simulink model "Braccio_trajectory_tracking_signal_based"  (R2021a)
settings: Solver=FixedStepAuto  StartTime=0.0  StopTime=inf  RelTol=1e-3  EnableMultiTasking=on
InitFcn:
  | cBase=90;
  | cShoulder=90;
  | cElbow=90;
  | cWristVer=90;
  | cWristRot=90;
  | cGripper=73;
undefined symbols (not defined in the file or in its folder): sigbuilder_block
libraries: arduinolib x7, simulink x1, sldrtlib x1
settings Model: SILPILModeSetting=veronly  ExtModeTrigDuration=2  Creator=loris  LastModifiedBy=loris
settings OptimizationCC: EnhancedBackFolding=on  PassReuseOutputArgsAs=Individual arguments  ZeroExternalMemoryAtStartup=off  ZeroInternalMemoryAtStartup=off  MaxStackSize=64  OptimizeBlockOrder=speed  DifferentSizesBufferReuse=on  OptimizationCustomize=off  EfficientTunableParamExpr=on
settings DebuggingCC: ParameterTunabilityLossMsg=error
settings HardwareCC: ProdBitPerInt=16  ProdBitPerPointer=16  ProdBitPerSizeT=16  ProdBitPerPtrDiffT=16  ProdLargestAtomicFloat=None  ProdWordSize=8  ProdHWDeviceType=Atmel->AVR
settings SFSimCC: MATLABDynamicMemAlloc=off
settings RTWCC: SystemTargetFile=ert.tlc  HardwareBoard=Arduino Mega 2560  TemplateMakefile=ert_default_tmf  Toolchain=Arduino AVR  BuildConfiguration=Faster Runs
settings CodeAppCC: ForceParamTrailComments=on  IgnoreCustomStorageClasses=off  OperatorAnnotations=on  SimulinkDataObjDesc=on  SFDataObjDesc=on  InsertBlockDesc=on
settings ERTTargetCC: SupportContinuousTime=on  SupportVariableSizeSignals=on  ExtModeStaticAllocSize=2048

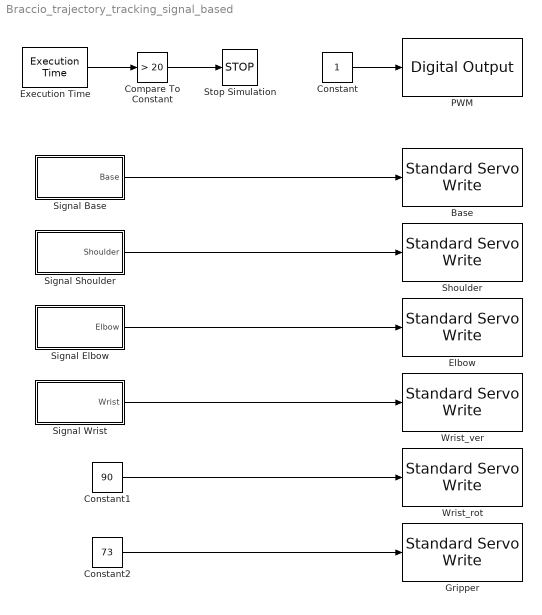
== system Braccio_trajectory_tracking_signal_based ==
  Base : arduinolib/Standard Servo Write  pinNumber=11  ServoIndex=0  blockPlatform=ARDUINO
  Compare To Constant : simulink/Logic and Bit Operations/Compare To Constant  relop=>  const=20  OutDataTypeStr=boolean
  Constant : Constant
  Constant1 : Constant  Value=90
  Constant2 : Constant  Value=73
  Elbow : arduinolib/Standard Servo Write  pinNumber=9  ServoIndex=1  blockPlatform=ARDUINO
  Execution Time : sldrtlib/Target Profiling/Execution Time  ShowTaskTimes=off
      settings: SourceProductBaseCode=WT
  Gripper : arduinolib/Standard Servo Write  pinNumber=3  ServoIndex=2  blockPlatform=ARDUINO
  PWM : arduinolib/Digital Output  pinNumber=12  Direction=output  blockPlatform=arduino
  Shoulder : arduinolib/Standard Servo Write  pinNumber=10  ServoIndex=3  blockPlatform=ARDUINO
  Signal Base : Subsystem  Tag=STV Subsys  LoadFcn=sigbuilder_block('load');  StartFcn=sigbuilder_block('start');  StopFcn=sigbuilder_block('stop');  ClipboardFcn=sigbuilder_block('clipboard');  mask(Sigbuilder block){tuvar=[0:10]}
      mask help: Simulink:masks:SigbuilderBlock_MD
      mask init:
      | if ~strcmp(get_param(bdroot(gcbh),'SimulationStatus'),'stopped') tuvar = sigbuilder_block('maskInit'); end
      settings: CopyFcn=sigbuilder_block('copy');  DeleteFcn=sigbuilder_block('delete');  ModelCloseFcn=sigbuilder_block('modelClose');  PreSaveFcn=sigbuilder_block('preSave');  PauseFcn=sigbuilder_block('pause');  ContinueFcn=sigbuilder_block('continue');  NameChangeFcn=sigbuilder_block('namechange');  OpenFcn=sigbuilder_block('open',[594 1310 550 349 ]);  CloseFcn=sigbuilder_block('close');
      mask Display: plot(0, 0, 100, 100,[2, 2, 32, 32, 2], [68, 8, 8, 68, 68],[32, 2], [38, 38], [32, 19, 2],[53, 60, 44], [32, 17, 17, 2],[16, 16, 31, 31]);txt = getActiveGroup(gcbh);text(2, 100, txt,'verticalAlignment', 'top');
  Signal Elbow : Subsystem  Tag=STV Subsys  LoadFcn=sigbuilder_block('load');  StartFcn=sigbuilder_block('start');  StopFcn=sigbuilder_block('stop');  ClipboardFcn=sigbuilder_block('clipboard');  mask(Sigbuilder block){tuvar=[0:10]}
      mask help: Simulink:masks:SigbuilderBlock_MD
      mask init:
      | if ~strcmp(get_param(bdroot(gcbh),'SimulationStatus'),'stopped') tuvar = sigbuilder_block('maskInit'); end
      settings: CopyFcn=sigbuilder_block('copy');  DeleteFcn=sigbuilder_block('delete');  ModelCloseFcn=sigbuilder_block('modelClose');  PreSaveFcn=sigbuilder_block('preSave');  PauseFcn=sigbuilder_block('pause');  ContinueFcn=sigbuilder_block('continue');  NameChangeFcn=sigbuilder_block('namechange');  OpenFcn=sigbuilder_block('open',[437.6 199.2 550.4 400 ]);  CloseFcn=sigbuilder_block('close');
      mask Display: plot(0, 0, 100, 100,[2, 2, 32, 32, 2], [68, 8, 8, 68, 68],[32, 2], [38, 38], [32, 19, 2],[53, 60, 44], [32, 17, 17, 2],[16, 16, 31, 31]);txt = getActiveGroup(gcbh);text(2, 100, txt,'verticalAlignment', 'top');
  Signal Shoulder : Subsystem  Tag=STV Subsys  LoadFcn=sigbuilder_block('load');  StartFcn=sigbuilder_block('start');  StopFcn=sigbuilder_block('stop');  ClipboardFcn=sigbuilder_block('clipboard');  mask(Sigbuilder block){tuvar=[0:10]}
      mask help: Simulink:masks:SigbuilderBlock_MD
      mask init:
      | if ~strcmp(get_param(bdroot(gcbh),'SimulationStatus'),'stopped') tuvar = sigbuilder_block('maskInit'); end
      settings: CopyFcn=sigbuilder_block('copy');  DeleteFcn=sigbuilder_block('delete');  ModelCloseFcn=sigbuilder_block('modelClose');  PreSaveFcn=sigbuilder_block('preSave');  PauseFcn=sigbuilder_block('pause');  ContinueFcn=sigbuilder_block('continue');  NameChangeFcn=sigbuilder_block('namechange');  OpenFcn=sigbuilder_block('open',[585 316 550 400 ]);  CloseFcn=sigbuilder_block('close');
      mask Display: plot(0, 0, 100, 100,[2, 2, 32, 32, 2], [68, 8, 8, 68, 68],[32, 2], [38, 38], [32, 19, 2],[53, 60, 44], [32, 17, 17, 2],[16, 16, 31, 31]);txt = getActiveGroup(gcbh);text(2, 100, txt,'verticalAlignment', 'top');
  Signal Wrist : Subsystem  Tag=STV Subsys  LoadFcn=sigbuilder_block('load');  StartFcn=sigbuilder_block('start');  StopFcn=sigbuilder_block('stop');  ClipboardFcn=sigbuilder_block('clipboard');  mask(Sigbuilder block){tuvar=[0:10]}
      mask help: Simulink:masks:SigbuilderBlock_MD
      mask init:
      | if ~strcmp(get_param(bdroot(gcbh),'SimulationStatus'),'stopped') tuvar = sigbuilder_block('maskInit'); end
      settings: CopyFcn=sigbuilder_block('copy');  DeleteFcn=sigbuilder_block('delete');  ModelCloseFcn=sigbuilder_block('modelClose');  PreSaveFcn=sigbuilder_block('preSave');  PauseFcn=sigbuilder_block('pause');  ContinueFcn=sigbuilder_block('continue');  NameChangeFcn=sigbuilder_block('namechange');  OpenFcn=sigbuilder_block('open',[437.6 199.2 550.4 400 ]);  CloseFcn=sigbuilder_block('close');
      mask Display: plot(0, 0, 100, 100,[2, 2, 32, 32, 2], [68, 8, 8, 68, 68],[32, 2], [38, 38], [32, 19, 2],[53, 60, 44], [32, 17, 17, 2],[16, 16, 31, 31]);txt = getActiveGroup(gcbh);text(2, 100, txt,'verticalAlignment', 'top');
  Stop Simulation : Stop
  Wrist_rot : arduinolib/Standard Servo Write  pinNumber=5  ServoIndex=4  blockPlatform=ARDUINO
  Wrist_ver : arduinolib/Standard Servo Write  pinNumber=6  ServoIndex=5  blockPlatform=ARDUINO
  wires:
  Constant/1 -> PWM/1
  Signal Base/1(Base) -> Base/1
  Signal Shoulder/1(Shoulder) -> Shoulder/1
  Signal Elbow/1(Elbow) -> Elbow/1
  Signal Wrist/1(Wrist) -> Wrist_ver/1
  Constant1/1 -> Wrist_rot/1
  Constant2/1 -> Gripper/1
  Execution Time/1 -> Compare To Constant/1
  Compare To Constant/1 -> Stop Simulation/1

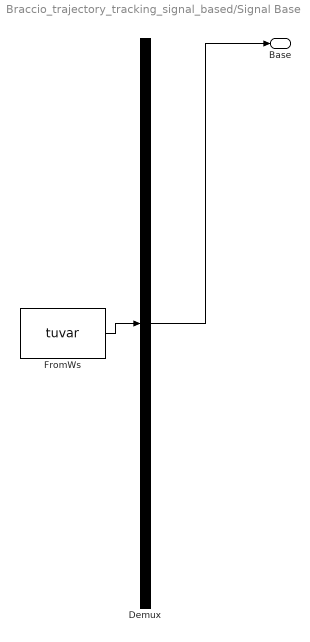
== system Braccio_trajectory_tracking_signal_based/Signal Base ==
  Demux : Demux  Tag=STV Demux  Outputs=1
      settings: DisplayOption=none
  FromWs : FromWorkspace  Tag=STV FromWs  VariableName=tuvar
      SigBuilderData=|
      | common.afterFinalStr = 'Extrapolate'
      | common.sampleTime = 0
      | dataSet.timeRange = [0 20]
      | dataSet.name = 'Group 1'
      | sbobj.Groups.Name = 'Group 1'
      | sbobj.Groups.Signals.Name = 'Base'
      | sbobj.Groups.Signals.XData = [0 0.2 0.4 0.6 0.8 1 1.2 1.4 1.6 1.8 2 2.2 2.4 2.6 2.8 3 3.2 3.4 3.6 3.8 4 4.2 4.4 4.6 4.8 5 5.2 5.4 5.6 5.8 6 6.2 6.4 6.6 6.8 7 7.2 7.4 7.6 7.8 8 8.2 8.4 8.6 8.8 9 9.2 9.4 9.6 9.8 10 10.2 10.4 10.6 10.8 11 11.2 11.4 11.6 11.8 12 12.2 12.4 12.6 12.8 13 13.2 13.4 13.6 13.8 14 14.2 14.4 14.6 14.8 15 15.2 15.4 15.6 15.8 16 16.2 16.4 16.6 16.8 17 17.2 17.4 17.6 17.8 18 18.2 18.4 18.6 18.8 19 19.2 19.4 19.6 19.8 20]
      | sbobj.Groups.Signals.YData = [90 90 1.13151518096 2.22402411518 3.28723976624 4.32060677531 5.32674779769 6.30802197271 7.26680517835 8.20541513658 9.12617137285 10.0314012612 10.9234295505 11.8046432279 12.6774581272 13.544405515 14.4080770144 15.2712272102 16.136772803 17.0078411564 17.8878192839 18.780412405 19.6897145122 20.6202941028 21.577299175 22.566586852 23.5948847099 24.6699931914 25.8010416489 26.9987776932 28.2739093645 29.6355594181 31.0934493562 32.658213992 34.3414915966 36.1559904427 38.115514386 40.2349251559 42.530009334 45.0172035073 47.7131424573 50.6339272404 53.7940681791 57.2050978124 60.8737501238 64.7998558727 68.9741248696 73.3761783447 77.9733299543 82.7206561007 87.5627548114 92.4372352396 97.2793346653 102.02666207 106.623815205 111.025870203 115.200140537 119.126247353 122.794900459 126.205930655 129.366071978 132.286852231 134.982792674 137.469990423 139.765074675 141.884485493 143.844009469 145.658508337 147.341785956 148.906550602 150.364440547 151.726090287 153.001221995 154.19895803 155.330006782 156.405115261 157.433413116 158.422700787 159.379705851 160.310285428 161.219587514 162.112179362 162.992158675 163.863226935 164.728772359 165.591922235 166.455593096 167.322533586 168.195354356 169.076564565 169.968593416 170.873820049 171.794571408 172.73317722 173.691938483 174.673186011 175.679231685 176.712394807 177.775011351 178.868516652 178.868516652]
      | sbobj.Groups.TimeRange = [0 20]
  Base : Outport  Tag=STV Outport
  wires:
  Demux/1 -> Base/1
  FromWs/1 -> Demux/1

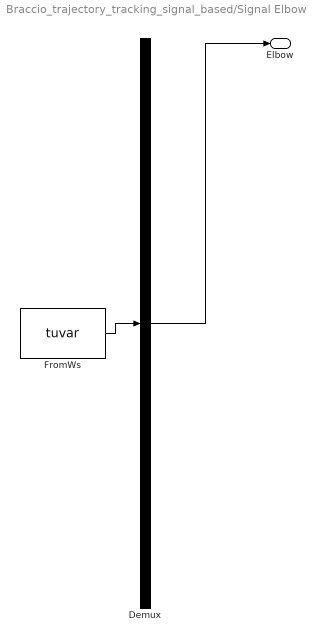
== system Braccio_trajectory_tracking_signal_based/Signal Elbow ==
  Demux : Demux  Tag=STV Demux  Outputs=1
      settings: DisplayOption=none
  FromWs : FromWorkspace  Tag=STV FromWs  VariableName=tuvar
      SigBuilderData=|
      | common.afterFinalStr = 'Extrapolate'
      | common.sampleTime = 0
      | dataSet.timeRange = [0 20]
      | dataSet.name = 'Group 1'
      | sbobj.Groups.Name = 'Group 1'
      | sbobj.Groups.Signals.Name = 'Elbow'
      | sbobj.Groups.Signals.XData = [0 0.2 0.4 0.6 0.8 1 1.2 1.4 1.6 1.8 2 2.2 2.4 2.6 2.8 3 3.2 3.4 3.6 3.8 4 4.2 4.4 4.6 4.8 5 5.2 5.4 5.6 5.8 6 6.2 6.4 6.6 6.8 7 7.2 7.4 7.6 7.8 8 8.2 8.4 8.6 8.8 9 9.2 9.4 9.6 9.8 10 10.2 10.4 10.6 10.8 11 11.2 11.4 11.6 11.8 12 12.2 12.4 12.6 12.8 13 13.2 13.4 13.6 13.8 14 14.2 14.4 14.6 14.8 15 15.2 15.4 15.6 15.8 16 16.2 16.4 16.6 16.8 17 17.2 17.4 17.6 17.8 18 18.2 18.4 18.6 18.8 19 19.2 19.4 19.6 19.8 20]
      | sbobj.Groups.Signals.YData = [90 90 85.869077391 81.9557081225 78.1686523913 74.4826588461 70.8868327406 67.375329246 63.9444920781 60.5918192687 57.3156144317 54.1150577978 50.9906470187 47.9449178507 44.9836136395 42.117049378 39.3614996263 36.7400228057 34.2820001173 32.0207689549 29.9892866353 28.2146272511 26.7128031796 25.4854397999 24.5191958887 23.787956617 23.2572158005 22.889880327 22.6528422779 22.5236791496 22.4885740621 22.5414436173 22.6920991248 22.9610428273 23.3732662577 23.9524703152 24.7160355452 25.6711096698 26.8122085019 28.1206383027 29.5657645601 31.1077754376 32.701130344 34.297857759 35.849963986 37.3106975436 38.6348209433 39.7783118336 40.6979712283 41.3513157787 41.6969460323 41.6969015947 41.3513994683 40.6988433788 39.7810942377 38.6410673081 37.322265596 35.8687628838 34.3254776983 32.7384064527 31.1543874152 29.6200060359 28.179472683 26.8716757954 25.7269963562 24.7646739994 23.9914351271 23.401788882 22.9800396687 22.703808567 22.5487500796 22.4941498829 22.5291094875 22.6579432691 22.892650643 23.254723348 23.7774612902 24.4992609059 25.4567840387 26.6786706184 28.1805154294 29.9620274343 32.0071658458 34.2874078319 36.7672986438 39.4106089505 42.1853464091 45.0665938597 48.0371231669 51.0865139498 54.2095466115 57.4045718105 60.672139464 64.01408397 67.4328952903 70.9314422299 74.5128589161 78.1806809842 81.9395150892 85.7992543201 89.5274796354]
      | sbobj.Groups.TimeRange = [0 20]
  Elbow : Outport  Tag=STV Outport
  wires:
  Demux/1 -> Elbow/1
  FromWs/1 -> Demux/1

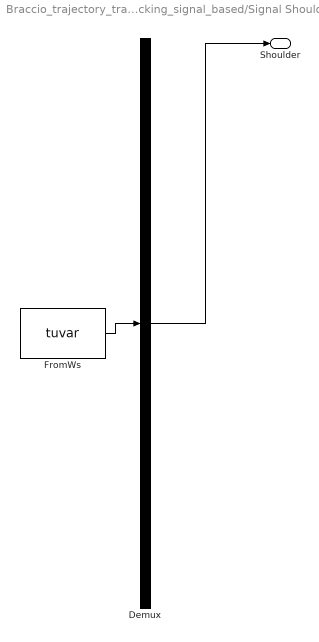
== system Braccio_trajectory_tracking_signal_based/Signal Shoulder ==
  Demux : Demux  Tag=STV Demux  Outputs=1
      settings: DisplayOption=none
  FromWs : FromWorkspace  Tag=STV FromWs  VariableName=tuvar
      SigBuilderData=|
      | common.afterFinalStr = 'Extrapolate'
      | common.sampleTime = 0
      | dataSet.timeRange = [0 20]
      | dataSet.name = 'Group 1'
      | sbobj.Groups.Name = 'Group 1'
      | sbobj.Groups.Signals.Name = 'Shoulder'
      | sbobj.Groups.Signals.XData = [0 0.2 0.4 0.6 0.8 1 1.2 1.4 1.6 1.8 2 2.2 2.4 2.6 2.8 3 3.2 3.4 3.6 3.8 4 4.2 4.4 4.6 4.8 5 5.2 5.4 5.6 5.8 6 6.2 6.4 6.6 6.8 7 7.2 7.4 7.6 7.8 8 8.2 8.4 8.6 8.8 9 9.2 9.4 9.6 9.8 10 10.2 10.4 10.6 10.8 11 11.2 11.4 11.6 11.8 12 12.2 12.4 12.6 12.8 13 13.2 13.4 13.6 13.8 14 14.2 14.4 14.6 14.8 15 15.2 15.4 15.6 15.8 16 16.2 16.4 16.6 16.8 17 17.2 17.4 17.6 17.8 18 18.2 18.4 18.6 18.8 19 19.2 19.4 19.6 19.8 20]
      | sbobj.Groups.Signals.YData = [90 90 93.8926166123 97.5629385566 101.015659732 104.229715418 107.177159639 109.825718824 112.139396418 114.078677377 115.601037937 116.662036219 117.217257293 117.225601928 116.653810503 115.482453152 113.712591473 111.371965406 108.518950768 105.242617958 101.658205416 97.89891246 94.1062417069 90.421348153 86.9789459963 83.9040099018 81.3105498925 79.3014056222 77.9681191271 77.3893223136 77.5843423025 78.4910877855 80.0298894139 82.1117088585 84.6401610814 87.513090625 90.6241491333 93.8648464216 97.1274771628 100.309103295 103.316437477 106.070891427 108.51306268 110.605520809 112.333497416 113.703383784 114.739453505 115.479362314 115.968857951 116.255868041 116.383882365 116.3839059 116.255821833 115.968381261 115.477826304 114.735956981 113.696803444 112.32261889 110.589260452 108.490759495 106.042605742 103.283152821 100.272738814 97.0905990177 93.830221725 90.5941572639 87.489249476 84.622878795 82.1003198186 80.0229405109 78.486788116 77.5810793441 77.3861526505 77.9651238027 79.2997692662 81.3120192577 83.9102741742 86.9909466528 90.4387032306 94.1269602865 97.9195605127 101.674561835 105.250657784 108.515816968 111.356577095 113.685709727 115.446277644 116.611332718 117.180008802 117.171443087 116.618331233 115.561143459 114.043676629 112.109854594 109.801856463 107.159050884 104.217685715 101.010960744 97.5692828336 93.9193817952 90.5151082155]
      | sbobj.Groups.TimeRange = [0 20]
  Shoulder : Outport  Tag=STV Outport
  wires:
  Demux/1 -> Shoulder/1
  FromWs/1 -> Demux/1

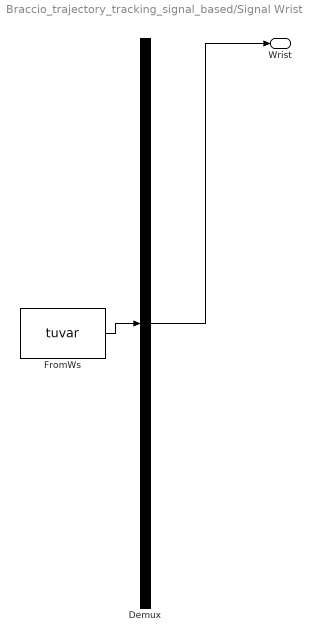
== system Braccio_trajectory_tracking_signal_based/Signal Wrist ==
  Demux : Demux  Tag=STV Demux  Outputs=1
      settings: DisplayOption=none
  FromWs : FromWorkspace  Tag=STV FromWs  VariableName=tuvar
      SigBuilderData=|
      | common.afterFinalStr = 'Extrapolate'
      | common.sampleTime = 0
      | dataSet.timeRange = [0 20]
      | dataSet.name = 'Group 1'
      | sbobj.Groups.Name = 'Group 1'
      | sbobj.Groups.Signals.Name = 'Wrist'
      | sbobj.Groups.Signals.XData = [0 0.2 0.4 0.6 0.8 1 1.2 1.4 1.6 1.8 2 2.2 2.4 2.6 2.8 3 3.2 3.4 3.6 3.8 4 4.2 4.4 4.6 4.8 5 5.2 5.4 5.6 5.8 6 6.2 6.4 6.6 6.8 7 7.2 7.4 7.6 7.8 8 8.2 8.4 8.6 8.8 9 9.2 9.4 9.6 9.8 10 10.2 10.4 10.6 10.8 11 11.2 11.4 11.6 11.8 12 12.2 12.4 12.6 12.8 13 13.2 13.4 13.6 13.8 14 14.2 14.4 14.6 14.8 15 15.2 15.4 15.6 15.8 16 16.2 16.4 16.6 16.8 17 17.2 17.4 17.6 17.8 18 18.2 18.4 18.6 18.8 19 19.2 19.4 19.6 19.8 20]
      | sbobj.Groups.Signals.YData = [90 90 83.2431486858 76.5809480588 70.0848725731 63.7780498933 57.6761513552 51.7956684763 46.1566121649 40.7840305569 35.7089167565 30.9687483649 26.6075962246 22.6752647777 19.2254301546 16.3119136007 13.9830503216 12.2741941602 11.1993131255 10.7434974672 10.8586185497 11.4638327593 12.4511339134 13.6944828529 15.060137958 16.4160510496 17.6391936541 18.620768378 19.2700014986 19.5179455129 19.3418427522 18.7760882183 17.8790068416 16.7247248487 15.3986492901 13.9933012631 12.6038316308 11.3227829539 10.2340494262 9.40648382386 8.88800570933 8.70140591676 8.8424701786 9.2809129371 9.96352339148 10.8187435083 11.7617788177 12.699667024 13.5361541724 14.1765787787 14.5331312932 14.5331664258 14.1765158101 13.535480664 12.6975112326 11.7569295022 10.8097440132 9.94886142689 9.25930326966 8.813193638 8.66462965309 8.8449842357 9.35952753049 10.1862720005 11.2775496307 12.564155167 13.9612591847 15.3750072032 16.7088607567 17.8691643526 18.7699161181 19.3371185456 19.5133387092 19.2657016347 18.6184444647 17.6412941043 16.4247947108 15.0766010413 13.7179414356 12.4788356895 11.4912905936 10.8803944095 10.7542919665 11.1950543558 12.252804625 13.944695926 16.2587416245 19.1609842112 22.6037467885 26.5332678152 30.8954820777 35.6398876987 40.7216259875 46.1024613511 51.7507795743 57.641286105 63.7543601639 70.0753586669 76.5935612709 83.2986162351 89.5374048785]
      | sbobj.Groups.TimeRange = [0 20]
  Wrist : Outport  Tag=STV Outport
  wires:
  Demux/1 -> Wrist/1
  FromWs/1 -> Demux/1
